simulink model "task8_8"  (R2021a)
settings: Solver=VariableStepAuto  StartTime=0.0  StopTime=10.0  RelTol=1e-3
settings Model: Creator=reemb  LastModifiedBy=reemb

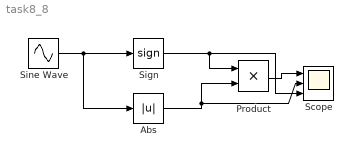
== system task8_8 ==
  Abs : Abs
  Product : Product
  Scope : Scope  NumInputPorts=3
  Sign : Signum
  Sine Wave : Sin  SampleTime=0
  wires:
  Sine Wave/1 -> Abs/1, Sign/1
  Sign/1 -> Scope/3, Product/1
  Abs/1 -> Scope/2, Product/2
  Product/1 -> Scope/1
